simulink model "MIMO_Case_A_MPC"  (R2024b)
settings: Solver=ode45  StartTime=0.0  StopTime=p.Tmax  FixedStep=p.Ts  RelTol=1e-3
values from neighbouring files (symbols this model uses):
  N = 4    [MIMO_Case_A_MPC_MHE_compensator.m]    (also in MIMO_Case_A_MPC_controller.m)
  nu = 2    [MHE_estimator.m]    (also in MIMO_Case_A_MPC_MHE_compensator.m; MIMO_Case_A_MPC_controller.m; MPC_controller.m)
  nx = 2    [MHE_estimator.m]    (also in MIMO_Case_A_MPC_MHE_compensator.m; MIMO_Case_A_MPC_controller.m; MPC_controller.m)
  p = MIMO_Case_A_params()    [MHE_estimator.m]    (also in MIMO_Case_A_MPC_MHE_compensator.m; MIMO_Case_A_MPC_controller.m; MPC_controller.m)
  phase_0 = 0    [MIMO_Case_A_MPC_MHE_compensator.m]    (also in MIMO_Case_A_MPC_controller.m)
  x_0 = [0 ... (first row only)    [MIMO_Case_A_MPC_MHE_compensator.m]    (also in MIMO_Case_A_MPC_controller.m)
undefined symbols (not defined in the file or in its folder): plecs
settings Model: Creator=rickd  LastModifiedBy=rickd

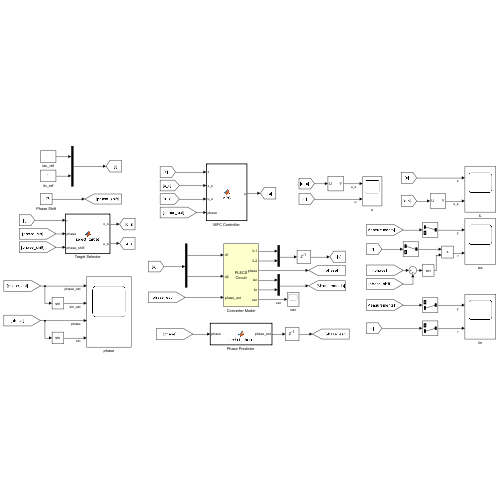
[thumbnail: Simulink's stored preview of the top-level diagram]
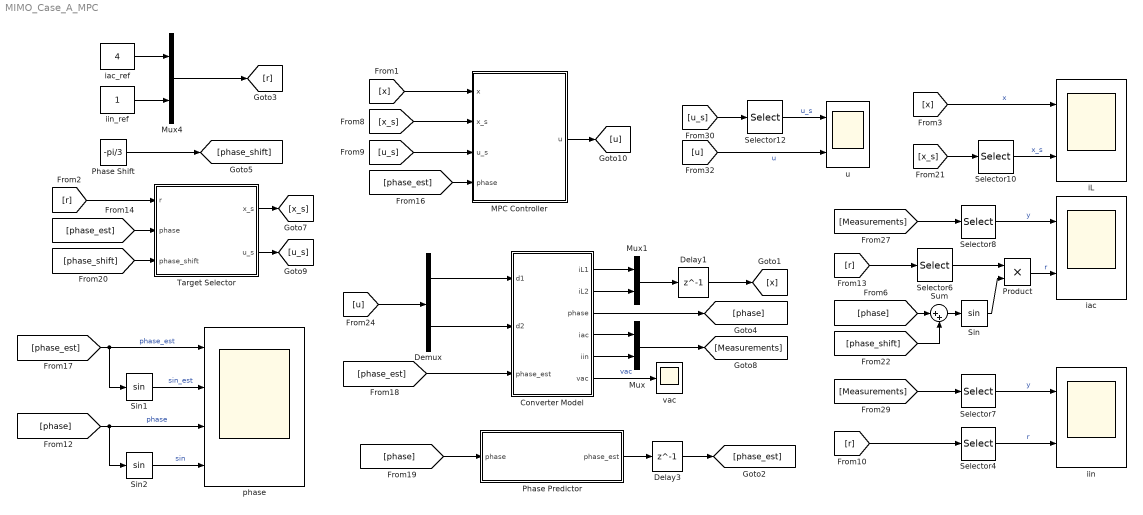
== system MIMO_Case_A_MPC ==
  Converter Model : Subsystem  LoadFcn=plecs('sl', 200);  InitFcn=plecs('sl', 214);  StartFcn=plecs('sl', 208);  StopFcn=plecs('sl', 209);  mask(PlecsCircuit){PLECSData=<binary blob, 11144 chars, not shown>}
      mask prompts: PLECSData "PLECS Data (Do not delete or modify!)"
      mask init:
      | % PLACE CUSTOM INITIALIZATIONS ABOVE
      | % DO NOT REMOVE
      | plecs('sl', 215);
      | % DO NOT REMOVE
      settings: CopyFcn=plecs('sl', 203);  DeleteFcn=plecs('sl', 205);  UndoDeleteFcn=plecs('sl', 206);  PreSaveFcn=plecs('sl', 211);  PostSaveFcn=plecs('sl', 201);  NameChangeFcn=plecs('sl', 210);  DestroyFcn=plecs('sl', 207);  PreCopyFcn=plecs('sl', 216);  OpenFcn=plecs('sl', 202);  ErrorFcn=plerrorfcn
      mask Help: eval('plecs(''help'', ''qthelp:///creatingacircuit.html'')')
      mask Display: disp('PLECS\nCircuit')
  Delay1 : Delay  DelayLength=1  InitialCondition=x_0  SampleTime=p.Ts
  Delay3 : Delay  DelayLength=1  InitialCondition=phase_0  SampleTime=p.Ts
  Demux : Demux  Outputs=nu
  MPC Controller : MATLAB Function  TreatAsAtomicUnit=on  SystemSampleTime=p.Ts
  Mux : Mux  Inputs=ny
  Mux1 : Mux  Inputs=nx
  Mux4 : Mux  Inputs=ny
  "Phase Predictor " : MATLAB Function  TreatAsAtomicUnit=on  SystemSampleTime=p.Ts
  Phase Shift : Constant  Value=-pi/3  SampleTime=p.Ts
  Product : Product
  Selector10 : Selector  InputPortWidth=(N+1)*nx  IndexOptions=Index vector (dialog)  Indices=[1:2]  OutputSizes=1
  Selector12 : Selector  InputPortWidth=(N+1)*nu  IndexOptions=Index vector (dialog)  Indices=[1:nu]  OutputSizes=1
  Selector4 : Selector  InputPortWidth=ny  IndexOptions=Index vector (dialog)  Indices=2  OutputSizes=1
  Selector6 : Selector  InputPortWidth=ny  IndexOptions=Index vector (dialog)  Indices=1  OutputSizes=1
  Selector7 : Selector  InputPortWidth=ny  IndexOptions=Index vector (dialog)  Indices=2  OutputSizes=1
  Selector8 : Selector  InputPortWidth=ny  IndexOptions=Index vector (dialog)  Indices=1  OutputSizes=1
  Sin : Trigonometry
  Sin1 : Trigonometry
  Sin2 : Trigonometry
  Sum : Sum  Inputs=|++
  Target Selector : MATLAB Function  TreatAsAtomicUnit=on  SystemSampleTime=p.Ts
  iL : Scope  NumInputPorts=2
  iac : Scope  NumInputPorts=2
  iac_ref : Constant  Value=4  SampleTime=p.Ts
  iin : Scope  NumInputPorts=2
  iin_ref : Constant  SampleTime=p.Ts
  phase : Scope  NumInputPorts=4
  u : Scope  NumInputPorts=2
  vac : Scope
  wires:
  MPC Controller/1(u) -> [u]
  [x_s] -> MPC Controller/2(x_s)
  [u_s] -> MPC Controller/3(u_s)
  Selector7/1 -> iin/1  "y"
  [x_s] -> Selector10/1
  Selector10/1 -> iL/2  "x_s"
  Demux/1 -> Converter Model/1(d1)
  Demux/2 -> Converter Model/2(d2)
  Target Selector/2(u_s) -> [u_s]
  Target Selector/1(x_s) -> [x_s]
  [u] -> Demux/1
  [u_s] -> Selector12/1
  Selector12/1 -> u/1  "u_s"
  Mux4/1 -> [r]
  [r] -> Target Selector/1(r)
  Selector4/1 -> iin/2  "r"
  [r] -> Selector4/1
  [x] -> MPC Controller/1(x)
  Mux/1 -> [Measurements]
  Selector8/1 -> iac/1  "y"
  [r] -> Selector6/1
  Converter Model/3(phase) -> [phase]
  [phase_est] -> phase/1, Sin1/1  "phase_est"
  iin_ref/1 -> Mux4/2
  [phase] -> "Phase Predictor "/1(phase)
  [phase_est] -> Target Selector/2(phase)
  iac_ref/1 -> Mux4/1
  Converter Model/4(iac) -> Mux/1
  Converter Model/5(iin) -> Mux/2
  [phase_est] -> MPC Controller/4(phase)
  [phase_est] -> Converter Model/3(phase_est)
  Selector6/1 -> Product/1
  Sin/1 -> Product/2
  Phase Shift/1 -> [phase_shift]
  [phase_shift] -> Target Selector/3(phase_shift)
  Product/1 -> iac/2  "r"
  Sum/1 -> Sin/1
  [phase_shift] -> Sum/2
  Sin1/1 -> phase/2  "sin_est"
  Sin2/1 -> phase/4  "sin"
  [phase] -> Sum/1
  [phase] -> Sin2/1, phase/3  "phase"
  "Phase Predictor "/1(phase_est) -> Delay3/1
  Delay3/1 -> [phase_est]
  [Measurements] -> Selector8/1
  [Measurements] -> Selector7/1
  [u] -> u/2  "u"
  Converter Model/1(iL1) -> Mux1/1
  Converter Model/2(iL2) -> Mux1/2
  Mux1/1 -> Delay1/1
  Delay1/1 -> [x]
  [x] -> iL/1  "x"
  Converter Model/6(vac) -> vac/1  "vac"

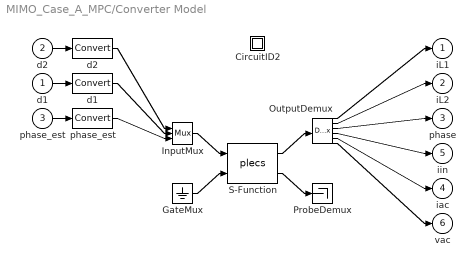
== system MIMO_Case_A_MPC/Converter Model ==
  d1 : Inport  PortDimensions=1
  d2 : Inport  Port=2  PortDimensions=1
  phase_est : Inport  Port=3  PortDimensions=1
  " CircuitID2 " : Subsystem
  " GateMux " : Ground
  " InputMux " : Mux  Inputs=[ 1 1 1 ]
  " OutputDemux " : Demux  Outputs=[ 1 1 1 1 1 1 ]
  " ProbeDemux " : Terminator
  " S-Function " : S-Function  FunctionName=plecs  SFunctionDeploymentMode=off  EnableBusSupport=off
  " d1 " : DataTypeConversion
  " d2 " : DataTypeConversion
  " phase_est " : DataTypeConversion
  iL1 : Outport  PortDimensions=1
  iL2 : Outport  Port=2  PortDimensions=1
  phase : Outport  Port=3  PortDimensions=1
  iac : Outport  Port=4  PortDimensions=1
  iin : Outport  Port=5  PortDimensions=1
  vac : Outport  Port=6  PortDimensions=1
  wires:
  " InputMux "/1 -> " S-Function "/1
  " GateMux "/1 -> " S-Function "/2
  " S-Function "/1 -> " OutputDemux "/1
  " S-Function "/2 -> " ProbeDemux "/1
  d2/1 -> " d2 "/1
  " d2 "/1 -> " InputMux "/1
  d1/1 -> " d1 "/1
  " d1 "/1 -> " InputMux "/2
  phase_est/1 -> " phase_est "/1
  " phase_est "/1 -> " InputMux "/3
  " OutputDemux "/1 -> iL1/1
  " OutputDemux "/2 -> iL2/1
  " OutputDemux "/3 -> phase/1
  " OutputDemux "/4 -> iin/1
  " OutputDemux "/5 -> iac/1
  " OutputDemux "/6 -> vac/1

== system MIMO_Case_A_MPC/Converter Model/ CircuitID2  ==

== matlab function MIMO_Case_A_MPC/Target Selector ==
  data: r input; phase input; phase_shift input; x_s output; u_s output; mpc parameter
function [x_s, u_s] = select_target(r, phase, phase_shift, mpc)

options = optimoptions('fsolve', 'Algorithm', 'levenberg-marquardt');

p = mpc.p;
f = @(x, u, phi) dynamics_wrapper(x, u, phi, p);
k1 = @(x, u, phi) f(x, u, phi);
k2 = @(x, u, phi) f(x + p.Ts/2*k1(x,u,phi), u, phi);
k3 = @(x, u, phi) f(x + p.Ts/2*k2(x,u,phi), u, phi);
k4 = @(x, u, phi) f(x + p.Ts*k3(x,u,phi), u, phi);
fd = @(x, u, phi) x + p.Ts/6*(k1(x,u,phi) + 2*k2(x,u,phi) + 2*k3(x,u,phi) + k4(x,u,phi));
gd = @(x, u, phi) output_wrapper(x, u, phi, p);

N = mpc.N;
nx = mpc.nx;
nu = mpc.nu;

persistent xu_0
if isempty(xu_0), xu_0 = zeros(nx+nu,1); end

persistent X_S U_S Iac_ref_old iin_ref_old phase_shift_old
if isempty(Iac_ref_old), Iac_ref_old = 0; end
if isempty(iin_ref_old), iin_ref_old = 0; end
if isempty(phase_shift_old), phase_shift_old = 0; end
if (isempty(X_S) && isempty(U_S)) || (Iac_ref_old ~= r(1)) || (iin_ref_old ~= r(2)) || (phase_shift_old ~= phase_shift)
    X_S = zeros((N+1)*nx, 1);
    U_S = zeros((N+1)*nu, 1);
    for k=1:N+1
        phase_k = mod(phase + 2*pi*p.fgrid*(k-1)*p.Ts, 2*pi);
        iac_ref = r(1) * sin(phase_k + phase_shift);
    
        fun = @(xu) [fd(xu(1:nx), xu(nx+1:nx+nu), phase_k); gd(xu(1:nx), xu(nx+1:nx+nu), phase_k)] - [xu(1:nx); [iac_ref; r(2)]];
    
        sol = fsolve(fun, xu_0, options);

        xu_0 = sol;

        X_S((k-1)*nx+1:k*nx,1) = sol(1:nx);
        U_S((k-1)*nu+1:k*nu,1) = sol(nx+1:nx+nu);
    end
else
    phase_N = mod(phase + 2*pi*p.fgrid*N*p.Ts, 2*pi);
    iac_ref = r(1) * sin(phase_N + phase_shift);

    fun = @(xu) [fd(xu(1:nx), xu(nx+1:nx+nu), phase_N); gd(xu(1:nx), xu(nx+1:nx+nu), phase_N)] - [xu(1:nx); [iac_ref; r(2)]];
    
    sol = fsolve(fun, xu_0, options);

    xu_0 = sol;
    
    solx = sol(1:nx);
    solu = sol(nx+1:nx+nu);
    
    X_S = [X_S(nx+1:end,1); solx];
    U_S = [U_S(nu+1:end,1); solu];
end

Iac_ref_old = r(1);
iin_ref_old = r(2);
phase_shift_old = phase_shift;

x_s = X_S;
u_s = U_S;

% Wrapper function to select the appropriate dynamics function
function xdot = dynamics_wrapper(x, u, phi, p)
    if phi <= pi
        [xdot, ~] = MIMO_Case_A_dynamics_SM1(x, u, phi, p);
    else
        [xdot, ~] = MIMO_Case_A_dynamics_SM2(x, u, phi, p);
    end
end

function y = output_wrapper(x, u, phi, p)
    if phi <= pi
        [~, y] = MIMO_Case_A_dynamics_SM1(x, u, phi, p);
    else
        [~, y] = MIMO_Case_A_dynamics_SM2(x, u, phi, p);
    end
end

end

== matlab function MIMO_Case_A_MPC/MPC Controller ==
  data: x input; x_s input; u_s input; phase input; u output; mpc parameter
function u = MPC(x, x_s, u_s, phase, mpc)

coder.extrinsic('fprintf');
options = optimoptions('fmincon', 'Algorithm', 'sqp');

p = mpc.p;
f = @(x, u, phi) dynamics_wrapper(x, u, phi, p);
k1 = @(x, u, phi) f(x, u, phi);
k2 = @(x, u, phi) f(x + p.Ts/2*k1(x,u,phi), u, phi);
k3 = @(x, u, phi) f(x + p.Ts/2*k2(x,u,phi), u, phi);
k4 = @(x, u, phi) f(x + p.Ts*k3(x,u,phi), u, phi);
fd = @(x, u, phi) x + p.Ts/6*(k1(x,u,phi) + 2*k2(x,u,phi) + 2*k3(x,u,phi) + k4(x,u,phi));

N = mpc.N;
nx = mpc.nx;
nu = mpc.nu;

if mod(phase + 2*pi*p.fgrid*N*p.Ts, 2*pi) <= pi
    Pf = mpc.Pinf1;
else
    Pf = mpc.Pinf2;
end
%Pf = zeros(nx, nx);
HxN = mpc.Hx;
hxN = mpc.hx;

Hessian = blkdiag(mpc.QX, Pf, mpc.RU);
fun = @(z) 1/2*((z - [x_s; u_s(1:end-nu,1)])' * Hessian * (z - [x_s; u_s(1:end-nu,1)]));
H = blkdiag(kron(eye(N), mpc.Hx), HxN, kron(eye(N), mpc.Hu));
h = [repmat(mpc.hx, N, 1);
     hxN;
     repmat(mpc.hu, N, 1)];
nonlcon = @(z) nlcon(z, fd, x, phase, nx, nu, N, p);

persistent z_0
if isempty(z_0), z_0 = mpc.z_0; end
[z, fval, exitflag, ~] = fmincon(fun, z_0, H, h, [], [], [], [], nonlcon, options);
u = z((N+1)*nx+1:(N+1)*nx+nu,1);
z_0 = z;

persistent iter max_fval
if isempty(iter), iter = 0; end
iter = iter + 1;
if isempty(max_fval), max_fval = 0; end
if fval > max_fval && iter > N+1
    max_fval = fval;
end
fprintf('Iteration: %d, ', iter)
fprintf('Cost: %f, ', fval)
fprintf('Worst-case cost: %f, ', max_fval)
fprintf('Exitflag: %f\n', exitflag)

function [c, ceq] = nlcon(z, f, x, phase, nx, nu, N, p)
    c = [];
    c1 = zeros(N*nx, 1); % Preallocate
    for i = 1:N
        c1((i-1)*nx+1:i*nx,1) = z(i*nx+1:(i+1)*nx,1) - f(z((i-1)*nx+1:i*nx,1), z((N+1)*nx+(i-1)*nu+1:(N+1)*nx+i*nu,1), mod(phase + 2*pi*p.fgrid*(i-1)*p.Ts, 2*pi));
    end
    ceq = [z(1:nx,1) - x; c1]; % Equality constraints
end

% Wrapper function to select the appropriate dynamics function
function xdot = dynamics_wrapper(x, u, phi, p)
    if phi <= pi
        [xdot, ~] = MIMO_Case_A_dynamics_SM1(x, u, phi, p);
    else
        [xdot, ~] = MIMO_Case_A_dynamics_SM2(x, u, phi, p);
    end
end

end

== matlab function MIMO_Case_A_MPC/Phase Predictor  ==
  data: phase input; phase_est output; p parameter
function phase_est = predict_phase(phase, p)
phase_est = mod(phase + 2*pi*p.fgrid*p.Ts, 2*pi);
end
